simulink model "Intergration"  (R2018b)
settings: Solver=FixedStepDiscrete  StartTime=0.0  StopTime=inf  FixedStep=0.005  RelTol=1e-3
PostLoadFcn:
  | if any(exist('dsrtsu_mdlpostloadfcn', 'file') ~= 0), dsrtsu_mdlpostloadfcn('Execute', bdroot); end
values from neighbouring files (symbols this model uses):
  P_x165_On = 1.0    [CAN_Tx.sldd]
  P_x242_On = 1.0    [CAN_Tx.sldd]
  P_x246_On = 1.0    [CAN_Tx.sldd]
libraries: rtican x112, simulink x59
(part 30 of 31)

== system Intergration/Radar410_RX/Subsystem41/Subsystem6 ==
  In1 : Inport
  Bus Creator : BusCreator  Inputs=20  OutDataTypeStr=Bus: Obj_Data  NonVirtualBus=on
      settings: InheritFromInputs=off
  Bus Selector : BusSelector  OutputSignals=FRS_P1_06_Msg_CheckSum,FRS_P1_06_Msg_AliveCounter,FRS_P1_06_Obj_ExstProb,FRS_P1_06_Obj_XVelRel_Stdev,FRS_P1_06_Obj_XAccRel,FRS_P1_06_Obj_ObstacleProb,FRS_P1_06_Obj_MotionPattern,FRS_P1_06_Obj_YPos_Stdev,FRS_P1_06_Obj_ValidFlag,FRS_P1_06_Obj_XPos_Stdev,FRS_P1_06_Obj_UpdateFlag,FRS_P1_06_Obj_ID,FRS_P2_06_Msg_CheckSum,FRS_P2_06_Msg_AliveCounter,FRS_P2_06_Obj_MeasFlag,FRS_P2_06_Obj_YVelRel,FRS_P2_06_Obj_Type,FRS_P2_06_Obj_XPos,FRS_P2_06_Obj_YPos,FRS_P2_06_Obj_XVelRel
  Data Type Conversion{,1..19} (20 alike) : DataTypeConversion  OutDataTypeStr=single
  Out1 : Outport  OutDataTypeStr=Bus: Obj_Data
  wires:
  Data Type Conversion19/1 -> Bus Creator/20
  Data Type Conversion14/1 -> Bus Creator/15
  Data Type Conversion8/1 -> Bus Creator/9
  Data Type Conversion7/1 -> Bus Creator/8
  Data Type Conversion3/1 -> Bus Creator/4
  Data Type Conversion4/1 -> Bus Creator/5
  Data Type Conversion1/1 -> Bus Creator/2
  Data Type Conversion13/1 -> Bus Creator/14
  Data Type Conversion2/1 -> Bus Creator/3
  Data Type Conversion/1 -> Bus Creator/1
  Bus Creator/1 -> Out1/1
  In1/1 -> Bus Selector/1
  Bus Selector/20 -> Data Type Conversion19/1  "<FRS_P2_06_Obj_XVelRel>"
  Bus Selector/18 -> Data Type Conversion17/1  "<FRS_P2_06_Obj_XPos>"
  Bus Selector/19 -> Data Type Conversion18/1  "<FRS_P2_06_Obj_YPos>"
  Bus Selector/14 -> Data Type Conversion13/1  "<FRS_P2_06_Msg_AliveCounter>"
  Data Type Conversion10/1 -> Bus Creator/11
  Bus Selector/10 -> Data Type Conversion9/1  "<FRS_P1_06_Obj_XPos_Stdev>"
  Bus Selector/17 -> Data Type Conversion16/1  "<FRS_P2_06_Obj_Type>"
  Bus Selector/9 -> Data Type Conversion8/1  "<FRS_P1_06_Obj_ValidFlag>"
  Data Type Conversion16/1 -> Bus Creator/17
  Bus Selector/12 -> Data Type Conversion11/1  "<FRS_P1_06_Obj_ID>"
  Data Type Conversion6/1 -> Bus Creator/7
  Bus Selector/16 -> Data Type Conversion15/1  "<FRS_P2_06_Obj_YVelRel>"
  Data Type Conversion17/1 -> Bus Creator/18
  Bus Selector/11 -> Data Type Conversion10/1  "<FRS_P1_06_Obj_UpdateFlag>"
  Data Type Conversion18/1 -> Bus Creator/19
  Bus Selector/6 -> Data Type Conversion5/1  "<FRS_P1_06_Obj_ObstacleProb>"
  Data Type Conversion9/1 -> Bus Creator/10
  Bus Selector/7 -> Data Type Conversion6/1  "<FRS_P1_06_Obj_MotionPattern>"
  Bus Selector/4 -> Data Type Conversion3/1  "<FRS_P1_06_Obj_XVelRel_Stdev>"
  Data Type Conversion5/1 -> Bus Creator/6
  Data Type Conversion11/1 -> Bus Creator/12
  Bus Selector/2 -> Data Type Conversion1/1  "<FRS_P1_06_Msg_AliveCounter>"
  Bus Selector/13 -> Data Type Conversion12/1  "<FRS_P2_06_Msg_CheckSum>"
  Bus Selector/3 -> Data Type Conversion2/1  "<FRS_P1_06_Obj_ExstProb>"
  Bus Selector/15 -> Data Type Conversion14/1  "<FRS_P2_06_Obj_MeasFlag>"
  Bus Selector/1 -> Data Type Conversion/1  "<FRS_P1_06_Msg_CheckSum>"
  Data Type Conversion15/1 -> Bus Creator/16
  Bus Selector/8 -> Data Type Conversion7/1  "<FRS_P1_06_Obj_YPos_Stdev>"
  Bus Selector/5 -> Data Type Conversion4/1  "<FRS_P1_06_Obj_XAccRel>"
  Data Type Conversion12/1 -> Bus Creator/13

== system Intergration/Radar410_RX/Subsystem41/Subsystem7 ==
  In1 : Inport
  Bus Creator : BusCreator  Inputs=20  OutDataTypeStr=Bus: Obj_Data  NonVirtualBus=on
      settings: InheritFromInputs=off
  Bus Selector : BusSelector  OutputSignals=FRS_P1_07_Msg_CheckSum,FRS_P1_07_Msg_AliveCounter,FRS_P1_07_Obj_ExstProb,FRS_P1_07_Obj_XVelRel_Stdev,FRS_P1_07_Obj_XAccRel,FRS_P1_07_Obj_ObstacleProb,FRS_P1_07_Obj_MotionPattern,FRS_P1_07_Obj_YPos_Stdev,FRS_P1_07_Obj_ValidFlag,FRS_P1_07_Obj_XPos_Stdev,FRS_P1_07_Obj_UpdateFlag,FRS_P1_07_Obj_ID,FRS_P2_07_Msg_CheckSum,FRS_P2_07_Msg_AliveCounter,FRS_P2_07_Obj_MeasFlag,FRS_P2_07_Obj_YVelRel,FRS_P2_07_Obj_Type,FRS_P2_07_Obj_XPos,FRS_P2_07_Obj_YPos,FRS_P2_07_Obj_XVelRel
  Data Type Conversion{,1..19} (20 alike) : DataTypeConversion  OutDataTypeStr=single
  Out1 : Outport  OutDataTypeStr=Bus: Obj_Data
  wires:
  Data Type Conversion12/1 -> Bus Creator/13
  Bus Selector/5 -> Data Type Conversion4/1  "<FRS_P1_07_Obj_XAccRel>"
  Bus Selector/8 -> Data Type Conversion7/1  "<FRS_P1_07_Obj_YPos_Stdev>"
  Data Type Conversion15/1 -> Bus Creator/16
  Bus Selector/1 -> Data Type Conversion/1  "<FRS_P1_07_Msg_CheckSum>"
  Bus Selector/15 -> Data Type Conversion14/1  "<FRS_P2_07_Obj_MeasFlag>"
  Bus Selector/3 -> Data Type Conversion2/1  "<FRS_P1_07_Obj_ExstProb>"
  Bus Selector/13 -> Data Type Conversion12/1  "<FRS_P2_07_Msg_CheckSum>"
  Bus Selector/2 -> Data Type Conversion1/1  "<FRS_P1_07_Msg_AliveCounter>"
  Data Type Conversion11/1 -> Bus Creator/12
  Data Type Conversion5/1 -> Bus Creator/6
  Bus Selector/4 -> Data Type Conversion3/1  "<FRS_P1_07_Obj_XVelRel_Stdev>"
  Bus Selector/7 -> Data Type Conversion6/1  "<FRS_P1_07_Obj_MotionPattern>"
  Data Type Conversion9/1 -> Bus Creator/10
  Bus Selector/6 -> Data Type Conversion5/1  "<FRS_P1_07_Obj_ObstacleProb>"
  Data Type Conversion18/1 -> Bus Creator/19
  Bus Selector/11 -> Data Type Conversion10/1  "<FRS_P1_07_Obj_UpdateFlag>"
  Data Type Conversion17/1 -> Bus Creator/18
  Bus Selector/16 -> Data Type Conversion15/1  "<FRS_P2_07_Obj_YVelRel>"
  Data Type Conversion6/1 -> Bus Creator/7
  Bus Selector/12 -> Data Type Conversion11/1  "<FRS_P1_07_Obj_ID>"
  Data Type Conversion16/1 -> Bus Creator/17
  Bus Selector/9 -> Data Type Conversion8/1  "<FRS_P1_07_Obj_ValidFlag>"
  Bus Selector/17 -> Data Type Conversion16/1  "<FRS_P2_07_Obj_Type>"
  Bus Selector/10 -> Data Type Conversion9/1  "<FRS_P1_07_Obj_XPos_Stdev>"
  Data Type Conversion10/1 -> Bus Creator/11
  Bus Selector/14 -> Data Type Conversion13/1  "<FRS_P2_07_Msg_AliveCounter>"
  Bus Selector/19 -> Data Type Conversion18/1  "<FRS_P2_07_Obj_YPos>"
  Bus Selector/18 -> Data Type Conversion17/1  "<FRS_P2_07_Obj_XPos>"
  Bus Selector/20 -> Data Type Conversion19/1  "<FRS_P2_07_Obj_XVelRel>"
  In1/1 -> Bus Selector/1
  Bus Creator/1 -> Out1/1
  Data Type Conversion/1 -> Bus Creator/1
  Data Type Conversion2/1 -> Bus Creator/3
  Data Type Conversion13/1 -> Bus Creator/14
  Data Type Conversion1/1 -> Bus Creator/2
  Data Type Conversion4/1 -> Bus Creator/5
  Data Type Conversion3/1 -> Bus Creator/4
  Data Type Conversion7/1 -> Bus Creator/8
  Data Type Conversion8/1 -> Bus Creator/9
  Data Type Conversion14/1 -> Bus Creator/15
  Data Type Conversion19/1 -> Bus Creator/20

== system Intergration/Radar410_RX/Subsystem41/Subsystem8 ==
  In1 : Inport
  Bus Creator : BusCreator  Inputs=20  OutDataTypeStr=Bus: Obj_Data  NonVirtualBus=on
      settings: InheritFromInputs=off
  Bus Selector : BusSelector  OutputSignals=FRS_P1_08_Msg_CheckSum,FRS_P1_08_Msg_AliveCounter,FRS_P1_08_Obj_ExstProb,FRS_P1_08_Obj_XVelRel_Stdev,FRS_P1_08_Obj_XAccRel,FRS_P1_08_Obj_ObstacleProb,FRS_P1_08_Obj_MotionPattern,FRS_P1_08_Obj_YPos_Stdev,FRS_P1_08_Obj_ValidFlag,FRS_P1_08_Obj_XPos_Stdev,FRS_P1_08_Obj_UpdateFlag,FRS_P1_08_Obj_ID,FRS_P2_08_Msg_CheckSum,FRS_P2_08_Msg_AliveCounter,FRS_P2_08_Obj_MeasFlag,FRS_P2_08_Obj_YVelRel,FRS_P2_08_Obj_Type,FRS_P2_08_Obj_XPos,FRS_P2_08_Obj_YPos,FRS_P2_08_Obj_XVelRel
  Data Type Conversion{,1..19} (20 alike) : DataTypeConversion  OutDataTypeStr=single
  Out1 : Outport  OutDataTypeStr=Bus: Obj_Data
  wires:
  Data Type Conversion12/1 -> Bus Creator/13
  Bus Selector/5 -> Data Type Conversion4/1  "<FRS_P1_08_Obj_XAccRel>"
  Bus Selector/8 -> Data Type Conversion7/1  "<FRS_P1_08_Obj_YPos_Stdev>"
  Data Type Conversion15/1 -> Bus Creator/16
  Bus Selector/1 -> Data Type Conversion/1  "<FRS_P1_08_Msg_CheckSum>"
  Bus Selector/15 -> Data Type Conversion14/1  "<FRS_P2_08_Obj_MeasFlag>"
  Bus Selector/3 -> Data Type Conversion2/1  "<FRS_P1_08_Obj_ExstProb>"
  Bus Selector/13 -> Data Type Conversion12/1  "<FRS_P2_08_Msg_CheckSum>"
  Bus Selector/2 -> Data Type Conversion1/1  "<FRS_P1_08_Msg_AliveCounter>"
  Data Type Conversion11/1 -> Bus Creator/12
  Data Type Conversion5/1 -> Bus Creator/6
  Bus Selector/4 -> Data Type Conversion3/1  "<FRS_P1_08_Obj_XVelRel_Stdev>"
  Bus Selector/7 -> Data Type Conversion6/1  "<FRS_P1_08_Obj_MotionPattern>"
  Data Type Conversion9/1 -> Bus Creator/10
  Bus Selector/6 -> Data Type Conversion5/1  "<FRS_P1_08_Obj_ObstacleProb>"
  Data Type Conversion18/1 -> Bus Creator/19
  Bus Selector/11 -> Data Type Conversion10/1  "<FRS_P1_08_Obj_UpdateFlag>"
  Data Type Conversion17/1 -> Bus Creator/18
  Bus Selector/16 -> Data Type Conversion15/1  "<FRS_P2_08_Obj_YVelRel>"
  Data Type Conversion6/1 -> Bus Creator/7
  Bus Selector/12 -> Data Type Conversion11/1  "<FRS_P1_08_Obj_ID>"
  Data Type Conversion16/1 -> Bus Creator/17
  Bus Selector/9 -> Data Type Conversion8/1  "<FRS_P1_08_Obj_ValidFlag>"
  Bus Selector/17 -> Data Type Conversion16/1  "<FRS_P2_08_Obj_Type>"
  Bus Selector/10 -> Data Type Conversion9/1  "<FRS_P1_08_Obj_XPos_Stdev>"
  Data Type Conversion10/1 -> Bus Creator/11
  Bus Selector/14 -> Data Type Conversion13/1  "<FRS_P2_08_Msg_AliveCounter>"
  Bus Selector/19 -> Data Type Conversion18/1  "<FRS_P2_08_Obj_YPos>"
  Bus Selector/18 -> Data Type Conversion17/1  "<FRS_P2_08_Obj_XPos>"
  Bus Selector/20 -> Data Type Conversion19/1  "<FRS_P2_08_Obj_XVelRel>"
  In1/1 -> Bus Selector/1
  Bus Creator/1 -> Out1/1
  Data Type Conversion/1 -> Bus Creator/1
  Data Type Conversion2/1 -> Bus Creator/3
  Data Type Conversion13/1 -> Bus Creator/14
  Data Type Conversion1/1 -> Bus Creator/2
  Data Type Conversion4/1 -> Bus Creator/5
  Data Type Conversion3/1 -> Bus Creator/4
  Data Type Conversion7/1 -> Bus Creator/8
  Data Type Conversion8/1 -> Bus Creator/9
  Data Type Conversion14/1 -> Bus Creator/15
  Data Type Conversion19/1 -> Bus Creator/20

== system Intergration/Radar410_RX/Subsystem41/Subsystem9 ==
  In1 : Inport
  Bus Creator : BusCreator  Inputs=20  OutDataTypeStr=Bus: Obj_Data  NonVirtualBus=on
      settings: InheritFromInputs=off
  Bus Selector : BusSelector  OutputSignals=FRS_P1_09_Msg_CheckSum,FRS_P1_09_Msg_AliveCounter,FRS_P1_09_Obj_ExstProb,FRS_P1_09_Obj_XVelRel_Stdev,FRS_P1_09_Obj_XAccRel,FRS_P1_09_Obj_ObstacleProb,FRS_P1_09_Obj_MotionPattern,FRS_P1_09_Obj_YPos_Stdev,FRS_P1_09_Obj_ValidFlag,FRS_P1_09_Obj_XPos_Stdev,FRS_P1_09_Obj_UpdateFlag,FRS_P1_09_Obj_ID,FRS_P2_09_Msg_CheckSum,FRS_P2_09_Msg_AliveCounter,FRS_P2_09_Obj_MeasFlag,FRS_P2_09_Obj_YVelRel,FRS_P2_09_Obj_Type,FRS_P2_09_Obj_XPos,FRS_P2_09_Obj_YPos,FRS_P2_09_Obj_XVelRel
  Data Type Conversion{,1..19} (20 alike) : DataTypeConversion  OutDataTypeStr=single
  Out1 : Outport  OutDataTypeStr=Bus: Obj_Data
  wires:
  Data Type Conversion19/1 -> Bus Creator/20
  Data Type Conversion14/1 -> Bus Creator/15
  Data Type Conversion8/1 -> Bus Creator/9
  Data Type Conversion7/1 -> Bus Creator/8
  Data Type Conversion3/1 -> Bus Creator/4
  Data Type Conversion4/1 -> Bus Creator/5
  Data Type Conversion1/1 -> Bus Creator/2
  Data Type Conversion13/1 -> Bus Creator/14
  Data Type Conversion2/1 -> Bus Creator/3
  Data Type Conversion/1 -> Bus Creator/1
  Bus Creator/1 -> Out1/1
  In1/1 -> Bus Selector/1
  Bus Selector/20 -> Data Type Conversion19/1  "<FRS_P2_09_Obj_XVelRel>"
  Bus Selector/18 -> Data Type Conversion17/1  "<FRS_P2_09_Obj_XPos>"
  Bus Selector/19 -> Data Type Conversion18/1  "<FRS_P2_09_Obj_YPos>"
  Bus Selector/14 -> Data Type Conversion13/1  "<FRS_P2_09_Msg_AliveCounter>"
  Data Type Conversion10/1 -> Bus Creator/11
  Bus Selector/10 -> Data Type Conversion9/1  "<FRS_P1_09_Obj_XPos_Stdev>"
  Bus Selector/17 -> Data Type Conversion16/1  "<FRS_P2_09_Obj_Type>"
  Bus Selector/9 -> Data Type Conversion8/1  "<FRS_P1_09_Obj_ValidFlag>"
  Data Type Conversion16/1 -> Bus Creator/17
  Bus Selector/12 -> Data Type Conversion11/1  "<FRS_P1_09_Obj_ID>"
  Data Type Conversion6/1 -> Bus Creator/7
  Bus Selector/16 -> Data Type Conversion15/1  "<FRS_P2_09_Obj_YVelRel>"
  Data Type Conversion17/1 -> Bus Creator/18
  Bus Selector/11 -> Data Type Conversion10/1  "<FRS_P1_09_Obj_UpdateFlag>"
  Data Type Conversion18/1 -> Bus Creator/19
  Bus Selector/6 -> Data Type Conversion5/1  "<FRS_P1_09_Obj_ObstacleProb>"
  Data Type Conversion9/1 -> Bus Creator/10
  Bus Selector/7 -> Data Type Conversion6/1  "<FRS_P1_09_Obj_MotionPattern>"
  Bus Selector/4 -> Data Type Conversion3/1  "<FRS_P1_09_Obj_XVelRel_Stdev>"
  Data Type Conversion5/1 -> Bus Creator/6
  Data Type Conversion11/1 -> Bus Creator/12
  Bus Selector/2 -> Data Type Conversion1/1  "<FRS_P1_09_Msg_AliveCounter>"
  Bus Selector/13 -> Data Type Conversion12/1  "<FRS_P2_09_Msg_CheckSum>"
  Bus Selector/3 -> Data Type Conversion2/1  "<FRS_P1_09_Obj_ExstProb>"
  Bus Selector/15 -> Data Type Conversion14/1  "<FRS_P2_09_Obj_MeasFlag>"
  Bus Selector/1 -> Data Type Conversion/1  "<FRS_P1_09_Msg_CheckSum>"
  Data Type Conversion15/1 -> Bus Creator/16
  Bus Selector/8 -> Data Type Conversion7/1  "<FRS_P1_09_Obj_YPos_Stdev>"
  Bus Selector/5 -> Data Type Conversion4/1  "<FRS_P1_09_Obj_XAccRel>"
  Data Type Conversion12/1 -> Bus Creator/13

== system Intergration/TX/Adapter_Tx/calc_0x165 ==
  <EngineTorqReq> : Inport
  <EngineTorqReqSt> : Inport  Port=2
  Bus Creator3 : BusCreator  Inputs=2  OutDataTypeStr=Bus: x165  NonVirtualBus=on
      settings: InheritFromInputs=off
  EngineTorqReq : Constant  Value=0  OutDataTypeStr=single
  EngineTorqReqSt : Constant  Value=0  OutDataTypeStr=boolean
  P_x165_On : Constant  Value=P_x165_On
  Switch : Switch  Criteria=u2 > Threshold  OutDataTypeStr=Inherit: Inherit via back propagation
  Switch1 : Switch  Criteria=u2 > Threshold  OutDataTypeStr=Inherit: Inherit via back propagation
  COM_x165_st : Outport
  wires:
  Switch1/1 -> Bus Creator3/2  "EngineTorqReq"
  P_x165_On/1 -> Switch/2, Switch1/2
  EngineTorqReq/1 -> Switch1/3
  <EngineTorqReq>/1 -> Switch1/1
  <EngineTorqReqSt>/1 -> Switch/1
  Switch/1 -> Bus Creator3/1  "EngineTorqReqSt"
  Bus Creator3/1 -> COM_x165_st/1  "COM_x165_st"
  EngineTorqReqSt/1 -> Switch/3

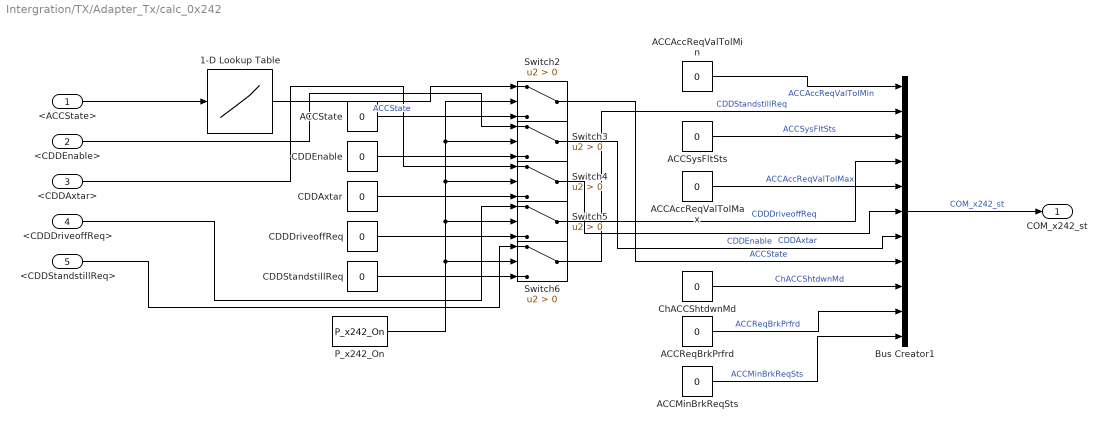
== system Intergration/TX/Adapter_Tx/calc_0x242 ==
  <ACCState> : Inport
  <CDDEnable> : Inport  Port=2
  <CDDAxtar> : Inport  Port=3
  <CDDDriveoffReq> : Inport  Port=4
  <CDDStandstillReq> : Inport  Port=5
  1-D Lookup Table : Lookup_n-D  NumberOfTableDimensions=1  BreakpointsForDimension1=[0,1,2,3,4]  Table=[0,1,2,5,3]  InternalRulePriority=Speed  RndMeth=Simplest  InputSameDT=on
  ACCAccReqValTolMax : Constant  Value=0  OutDataTypeStr=single
  ACCAccReqValTolMin : Constant  Value=0  OutDataTypeStr=single
  ACCMinBrkReqSts : Constant  Value=0  OutDataTypeStr=boolean
  ACCReqBrkPrfrd : Constant  Value=0  OutDataTypeStr=boolean
  ACCState : Constant  Value=0  OutDataTypeStr=single
  ACCSysFltSts : Constant  Value=0  OutDataTypeStr=single
  Bus Creator1 : BusCreator  Inputs=11  OutDataTypeStr=Bus: x242  NonVirtualBus=on
  CDDAxtar : Constant  Value=0  OutDataTypeStr=single
  CDDDriveoffReq : Constant  Value=0  OutDataTypeStr=boolean
  CDDEnable : Constant  Value=0  OutDataTypeStr=boolean
  CDDStandstillReq : Constant  Value=0  OutDataTypeStr=boolean
  ChACCShtdwnMd : Constant  Value=0  OutDataTypeStr=single
  P_x242_On : Constant  Value=P_x242_On
  Switch{2..6} (5 alike) : Switch  Criteria=u2 > Threshold  OutDataTypeStr=Inherit: Inherit via back propagation
  COM_x242_st : Outport
  wires:
  Switch2/1 -> Bus Creator1/8  "ACCState"
  CDDStandstillReq/1 -> Switch6/3
  ACCState/1 -> Switch2/3
  <CDDStandstillReq>/1 -> Switch6/1
  P_x242_On/1 -> Switch5/2, Switch4/2, Switch2/2, Switch3/2, Switch6/2
  CDDDriveoffReq/1 -> Switch5/3
  ACCAccReqValTolMax/1 -> Bus Creator1/5  "ACCAccReqValTolMax"
  CDDAxtar/1 -> Switch4/3
  CDDEnable/1 -> Switch3/3
  <ACCState>/1 -> 1-D Lookup Table/1
  Switch3/1 -> Bus Creator1/7  "CDDEnable"
  ACCReqBrkPrfrd/1 -> Bus Creator1/10  "ACCReqBrkPrfrd"
  ChACCShtdwnMd/1 -> Bus Creator1/9  "ChACCShtdwnMd"
  Switch4/1 -> Bus Creator1/6  "CDDAxtar"
  Switch6/1 -> Bus Creator1/2  "CDDStandstillReq"
  ACCSysFltSts/1 -> Bus Creator1/3  "ACCSysFltSts"
  ACCMinBrkReqSts/1 -> Bus Creator1/11  "ACCMinBrkReqSts"
  Switch5/1 -> Bus Creator1/4  "CDDDriveoffReq"
  <CDDDriveoffReq>/1 -> Switch5/1
  ACCAccReqValTolMin/1 -> Bus Creator1/1  "ACCAccReqValTolMin"
  1-D Lookup Table/1 -> Switch2/1  "ACCState"
  Bus Creator1/1 -> COM_x242_st/1  "COM_x242_st"
  <CDDAxtar>/1 -> Switch4/1
  <CDDEnable>/1 -> Switch3/1

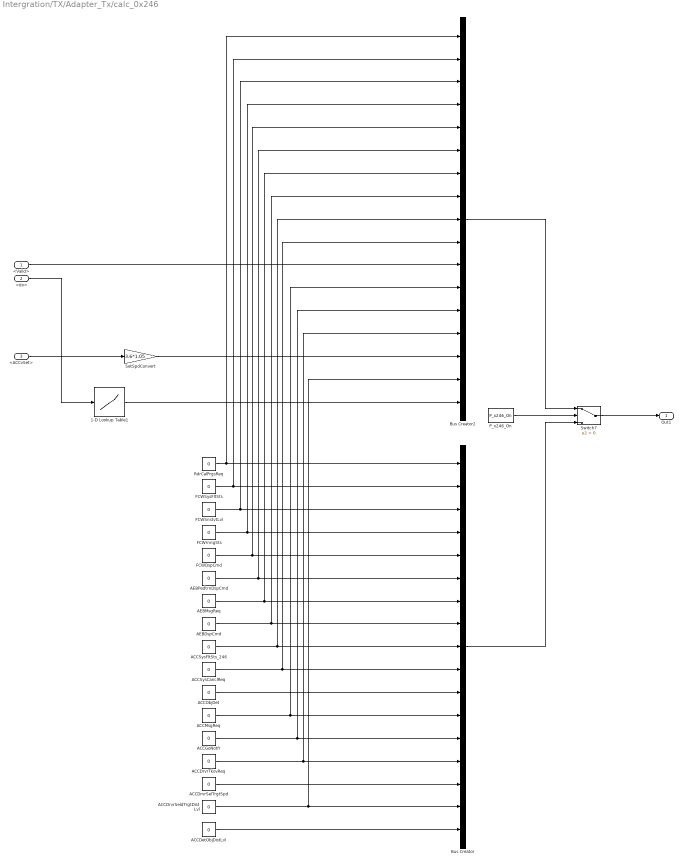
== system Intergration/TX/Adapter_Tx/calc_0x246 ==
  <Valid> : Inport
  <dx> : Inport  Port=2
  <ACCvSet> : Inport  Port=3
  1-D Lookup Table1 : Lookup_n-D  NumberOfTableDimensions=1  LookupTableObject=''  BreakpointsForDimension1=[5,10,20,30,40]  BreakpointsForDimension1FirstPoint=10  BreakpointsForDimension2FirstPoint=10  BreakpointsForDimension1Spacing=12  BreakpointsForDimension2Spacing=12  IndexSearchMethod=Linear search  Table=[1,2,3,4,5]  InterpMethod=Flat  InternalRulePriority=Speed  RndMeth=Simplest  InputSameDT=on
  ACCDetObjDistLvl : Constant  Value=0  OutDataTypeStr=single
  ACCDrvrSelTrgtSpd : Constant  Value=0  OutDataTypeStr=single
  ACCDrvrSeldTrgtDistLvl : Constant  Value=0  OutDataTypeStr=single
  ACCDrvrTkovReq : Constant  Value=0  OutDataTypeStr=boolean
  ACCGoNotfr : Constant  Value=0  OutDataTypeStr=boolean
  ACCMsgReq : Constant  Value=0  OutDataTypeStr=single
  ACCObjDet : Constant  Value=0  OutDataTypeStr=boolean
  ACCSysCanclReq : Constant  Value=0  OutDataTypeStr=single
  ACCSysFltSts_246 : Constant  Value=0  OutDataTypeStr=single
  AEBDspCmd : Constant  Value=0  OutDataTypeStr=single
  AEBMsgReq : Constant  Value=0  OutDataTypeStr=single
  AEBPedtrnDspCmd : Constant  Value=0  OutDataTypeStr=single
  Bus Creator : BusCreator  Inputs=17  OutDataTypeStr=Bus: x246  NonVirtualBus=on
      settings: InheritFromInputs=off
  Bus Creator2 : BusCreator  Inputs=17  OutDataTypeStr=Bus: x246  NonVirtualBus=on
      settings: InheritFromInputs=off
  FCWDspCmd : Constant  Value=0  OutDataTypeStr=single
  FCWSnstvtLvl : Constant  Value=0  OutDataTypeStr=single
  FCWSysFltSts : Constant  Value=0  OutDataTypeStr=single
  FCWrnngSts : Constant  Value=0  OutDataTypeStr=single
  P_x246_On : Constant  Value=P_x246_On
  RdrCalPrgsReq : Constant  Value=0  OutDataTypeStr=single
  SetSpdConvert : Gain  Gain=3.6*1.05
  Switch7 : Switch  Criteria=u2 > Threshold
  Out1 : Outport
  wires:
  ACCDrvrSeldTrgtDistLvl/1 -> Bus Creator2/16, Bus Creator/16
  ACCSysCanclReq/1 -> Bus Creator2/10, Bus Creator/10
  FCWDspCmd/1 -> Bus Creator2/5, Bus Creator/5
  ACCSysFltSts_246/1 -> Bus Creator2/9, Bus Creator/9
  FCWrnngSts/1 -> Bus Creator2/4, Bus Creator/4
  SetSpdConvert/1 -> Bus Creator2/15
  Bus Creator2/1 -> Switch7/1
  Bus Creator/1 -> Switch7/3
  ACCDetObjDistLvl/1 -> Bus Creator/17
  <ACCvSet>/1 -> SetSpdConvert/1
  FCWSysFltSts/1 -> Bus Creator2/2, Bus Creator/2
  RdrCalPrgsReq/1 -> Bus Creator2/1, Bus Creator/1
  ACCGoNotfr/1 -> Bus Creator2/13, Bus Creator/13
  ACCDrvrSelTrgtSpd/1 -> Bus Creator/15
  <Valid>/1 -> Bus Creator2/11
  AEBMsgReq/1 -> Bus Creator2/7, Bus Creator/7
  AEBDspCmd/1 -> Bus Creator2/8, Bus Creator/8
  ACCDrvrTkovReq/1 -> Bus Creator2/14, Bus Creator/14
  <dx>/1 -> 1-D Lookup Table1/1
  FCWSnstvtLvl/1 -> Bus Creator2/3, Bus Creator/3
  ACCMsgReq/1 -> Bus Creator2/12, Bus Creator/12
  ACCObjDet/1 -> Bus Creator/11
  P_x246_On/1 -> Switch7/2
  AEBPedtrnDspCmd/1 -> Bus Creator2/6, Bus Creator/6
  1-D Lookup Table1/1 -> Bus Creator2/17
  Switch7/1 -> Out1/1

== system Intergration/TX/Adapter_Tx/calc_0x255 ==
  ACCvSet : Inport
  ACCState : Inport  Port=2
  dx : Inport  Port=3
  dy : Inport  Port=4
  Type : Inport  Port=5
  ACC_Error : Constant  Value=0  OutDataTypeStr=single
  ACC_Passive_Res : Constant  Value=0  OutDataTypeStr=single
  ACC_Tip : Constant  Value=0  OutDataTypeStr=single
  Bus Creator : BusCreator  Inputs=9  OutDataTypeStr=Bus: x255  NonVirtualBus=on
      settings: InheritFromInputs=off
  TimeGapRes : Constant  Value=0  OutDataTypeStr=single
  Out1 : Outport
  wires:
  dy/1 -> Bus Creator/1
  dx/1 -> Bus Creator/2
  Type/1 -> Bus Creator/3
  ACC_Tip/1 -> Bus Creator/4
  ACCState/1 -> Bus Creator/5
  ACC_Passive_Res/1 -> Bus Creator/6
  ACC_Error/1 -> Bus Creator/7
  TimeGapRes/1 -> Bus Creator/8
  ACCvSet/1 -> Bus Creator/9
  Bus Creator/1 -> Out1/1

== system Intergration/TX/ESC_DA_MESSAGE_0x127/RollingCounter1 ==
  Add2 : Sum
  Constant5 : Constant
  Constant6 : Constant  Value=-1
  Delay : Delay  DelayLength=1
  Switch : Switch  Criteria=u2 > Threshold  Threshold=14
  RC : Outport
  wires:
  Constant6/1 -> Switch/1
  Switch/1 -> Add2/2
  Delay/1 -> RC/1, Switch/3, Switch/2
  Add2/1 -> Delay/1
  Constant5/1 -> Add2/1

== system Intergration/TX/ESC_DA_MESSAGE_0x127/Subsystem ==
  NoBrakeForce : Inport
  ABP_available : Inport  Port=2
  AEB_available : Inport  Port=3
  Add : Sum  Inputs=+++
  Bitwise Operator1 : simulink/Logic and Bit Operations/Bitwise Operator  logicop=AND  UseBitMask=on  BitMask=bin2dec('00010000')  BitMaskRealWorld=Stored Integer
  Bitwise Operator2 : simulink/Logic and Bit Operations/Bitwise Operator  logicop=AND  UseBitMask=on  BitMask=bin2dec('00000100')  BitMaskRealWorld=Stored Integer
  Bitwise Operator3 : simulink/Logic and Bit Operations/Bitwise Operator  logicop=AND  UseBitMask=on  BitMask=bin2dec('10000000')  BitMaskRealWorld=Stored Integer
  Data Type Conversion1 : DataTypeConversion  OutDataTypeStr=uint8
  Data Type Conversion2 : DataTypeConversion  OutDataTypeStr=uint8
  Data Type Conversion3 : DataTypeConversion  OutDataTypeStr=uint8
  Shift Arithmetic1 : ArithShift  BitShiftNumber=4  BitShiftDirection=Left
  Shift Arithmetic2 : ArithShift  BitShiftNumber=7  BitShiftDirection=Left
  Shift Arithmetic3 : ArithShift  BitShiftNumber=2  BitShiftDirection=Left
  Byte0 : Outport
  wires:
  Bitwise Operator1/1 -> Add/2
  Data Type Conversion2/1 -> Shift Arithmetic3/1
  Shift Arithmetic2/1 -> Bitwise Operator3/1
  Data Type Conversion3/1 -> Shift Arithmetic2/1
  Data Type Conversion1/1 -> Shift Arithmetic1/1
  Shift Arithmetic3/1 -> Bitwise Operator2/1
  Bitwise Operator3/1 -> Add/1
  Add/1 -> Byte0/1
  Shift Arithmetic1/1 -> Bitwise Operator1/1
  Bitwise Operator2/1 -> Add/3
  NoBrakeForce/1 -> Data Type Conversion2/1
  ABP_available/1 -> Data Type Conversion1/1
  AEB_available/1 -> Data Type Conversion3/1

== system Intergration/TX/ESC_DA_MESSAGE_0x127/Subsystem1 ==
  ABA_available : Inport
  AWB_available : Inport  Port=2
  VehSdslStsHSC2 : Inport  Port=3
  Add : Sum  Inputs=+++
  Bitwise Operator1 : simulink/Logic and Bit Operations/Bitwise Operator  logicop=AND  UseBitMask=on  BitMask=bin2dec('00001000')  BitMaskRealWorld=Stored Integer
  Bitwise Operator2 : simulink/Logic and Bit Operations/Bitwise Operator  logicop=AND  UseBitMask=on  BitMask=bin2dec('11000000')  BitMaskRealWorld=Stored Integer
  Bitwise Operator3 : simulink/Logic and Bit Operations/Bitwise Operator  logicop=AND  UseBitMask=on  BitMask=bin2dec('00000010')  BitMaskRealWorld=Stored Integer
  Data Type Conversion1 : DataTypeConversion  OutDataTypeStr=uint8
  Data Type Conversion2 : DataTypeConversion  OutDataTypeStr=uint8
  Data Type Conversion3 : DataTypeConversion  OutDataTypeStr=uint8
  Shift Arithmetic1 : ArithShift  BitShiftNumber=3  BitShiftDirection=Left
  Shift Arithmetic2 : ArithShift  BitShiftNumber=1  BitShiftDirection=Left
  Shift Arithmetic3 : ArithShift  BitShiftNumber=6  BitShiftDirection=Left
  Byte1 : Outport
  wires:
  Shift Arithmetic3/1 -> Bitwise Operator2/1
  Shift Arithmetic1/1 -> Bitwise Operator1/1
  ABA_available/1 -> Data Type Conversion3/1
  VehSdslStsHSC2/1 -> Data Type Conversion2/1
  Bitwise Operator1/1 -> Add/2
  Data Type Conversion3/1 -> Shift Arithmetic2/1
  Shift Arithmetic2/1 -> Bitwise Operator3/1
  Bitwise Operator2/1 -> Add/1
  Data Type Conversion1/1 -> Shift Arithmetic1/1
  Data Type Conversion2/1 -> Shift Arithmetic3/1
  Bitwise Operator3/1 -> Add/3
  Add/1 -> Byte1/1
  AWB_available/1 -> Data Type Conversion1/1

== system Intergration/TX/ESC_DA_MESSAGE_0x127/Subsystem2 ==
  In1 : Inport
  Bitwise Operator2 : simulink/Logic and Bit Operations/Bitwise Operator  logicop=AND  UseBitMask=on  BitMask=bin2dec('00001111')  BitMaskRealWorld=Stored Integer
  Data Type Conversion1 : DataTypeConversion  OutDataTypeStr=uint8
  Byte6 : Outport
  wires:
  In1/1 -> Data Type Conversion1/1
  Bitwise Operator2/1 -> Byte6/1
  Data Type Conversion1/1 -> Bitwise Operator2/1

== system Intergration/TX/ESC_FrontWheelSpeedKPH_0x123/RollingCounter1 ==
  Add2 : Sum
  Constant5 : Constant
  Constant6 : Constant  Value=-1
  Delay : Delay  DelayLength=1
  Switch : Switch  Criteria=u2 > Threshold  Threshold=14
  RC : Outport
  wires:
  Constant6/1 -> Switch/1
  Switch/1 -> Add2/2
  Delay/1 -> RC/1, Switch/3, Switch/2
  Add2/1 -> Delay/1
  Constant5/1 -> Add2/1

== system Intergration/TX/ESC_FrontWheelSpeedKPH_0x123/Subsystem ==
  <WhlGndVelLDrvn_Radar> : Inport
  Bitwise Operator1 : simulink/Logic and Bit Operations/Bitwise Operator  logicop=AND  UseBitMask=on  BitMask=bin2dec('11111111')  BitMaskRealWorld=Stored Integer
  Constant : Constant  Value=0.05625
  Constant1 : Constant  Value=0.05625
  Data Type Conversion1 : DataTypeConversion  OutDataTypeStr=uint16
  Data Type Conversion2 : DataTypeConversion  OutDataTypeStr=uint8
  Divide : Product  Inputs=*/
  Multiply : Product
  Shift Arithmetic1 : ArithShift  BitShiftNumber=5  BitShiftDirection=Right
  Out1 : Outport
  Byte0 : Outport  Port=2
  Output : Outport  Port=3
  wires:
  Bitwise Operator1/1 -> Data Type Conversion2/1
  Shift Arithmetic1/1 -> Bitwise Operator1/1
  Divide/1 -> Data Type Conversion1/1
  Constant/1 -> Divide/2
  Constant1/1 -> Multiply/1
  Data Type Conversion1/1 -> Output/1, Multiply/2, Shift Arithmetic1/1
  <WhlGndVelLDrvn_Radar>/1 -> Divide/1
  Multiply/1 -> Out1/1
  Data Type Conversion2/1 -> Byte0/1

== system Intergration/TX/ESC_FrontWheelSpeedKPH_0x123/Subsystem1 ==
  In1 : Inport
  <LDrvnWhlRotlDircn> : Inport  Port=2
  Add : Sum
  Bitwise Operator1 : simulink/Logic and Bit Operations/Bitwise Operator  logicop=AND  UseBitMask=on  BitMask=bin2dec('00000110')  BitMaskRealWorld=Stored Integer
  Bitwise Operator2 : simulink/Logic and Bit Operations/Bitwise Operator  logicop=AND  UseBitMask=on  BitMask=bin2dec('11111000')  BitMaskRealWorld=Stored Integer
  Data Type Conversion1 : DataTypeConversion  OutDataTypeStr=uint8
  Data Type Conversion2 : DataTypeConversion  OutDataTypeStr=uint8
  Shift Arithmetic1 : ArithShift  BitShiftNumber=1  BitShiftDirection=Left
  Shift Arithmetic2 : ArithShift  BitShiftNumber=3  BitShiftDirection=Left
  Byte1 : Outport
  wires:
  <LDrvnWhlRotlDircn>/1 -> Data Type Conversion1/1
  Bitwise Operator2/1 -> Data Type Conversion2/1
  Data Type Conversion1/1 -> Shift Arithmetic1/1
  Bitwise Operator1/1 -> Add/1
  Shift Arithmetic1/1 -> Bitwise Operator1/1
  Add/1 -> Byte1/1
  Shift Arithmetic2/1 -> Bitwise Operator2/1
  In1/1 -> Shift Arithmetic2/1
  Data Type Conversion2/1 -> Add/2

== system Intergration/TX/ESC_FrontWheelSpeedKPH_0x123/Subsystem2 ==
  <WhlGndVelLDrvn_Radar> : Inport
  Bitwise Operator1 : simulink/Logic and Bit Operations/Bitwise Operator  logicop=AND  UseBitMask=on  BitMask=bin2dec('11111111')  BitMaskRealWorld=Stored Integer
  Constant : Constant  Value=0.05625
  Constant1 : Constant  Value=0.05625
  Data Type Conversion1 : DataTypeConversion  OutDataTypeStr=uint16
  Data Type Conversion2 : DataTypeConversion  OutDataTypeStr=uint8
  Divide : Product  Inputs=*/
  Multiply : Product
  Shift Arithmetic1 : ArithShift  BitShiftNumber=5  BitShiftDirection=Right
  Out1 : Outport
  Byte2 : Outport  Port=2
  Output : Outport  Port=3
  wires:
  Bitwise Operator1/1 -> Data Type Conversion2/1
  Shift Arithmetic1/1 -> Bitwise Operator1/1
  Divide/1 -> Data Type Conversion1/1
  Constant/1 -> Divide/2
  Constant1/1 -> Multiply/1
  Data Type Conversion1/1 -> Output/1, Multiply/2, Shift Arithmetic1/1
  <WhlGndVelLDrvn_Radar>/1 -> Divide/1
  Multiply/1 -> Out1/1
  Data Type Conversion2/1 -> Byte2/1

== system Intergration/TX/ESC_FrontWheelSpeedKPH_0x123/Subsystem3 ==
  In1 : Inport
  <LDrvnWhlRotlDircn> : Inport  Port=2
  Add : Sum
  Bitwise Operator1 : simulink/Logic and Bit Operations/Bitwise Operator  logicop=AND  UseBitMask=on  BitMask=bin2dec('00000110')  BitMaskRealWorld=Stored Integer
  Bitwise Operator2 : simulink/Logic and Bit Operations/Bitwise Operator  logicop=AND  UseBitMask=on  BitMask=bin2dec('11111000')  BitMaskRealWorld=Stored Integer
  Data Type Conversion1 : DataTypeConversion  OutDataTypeStr=uint8
  Data Type Conversion2 : DataTypeConversion  OutDataTypeStr=uint8
  Shift Arithmetic1 : ArithShift  BitShiftNumber=1  BitShiftDirection=Left
  Shift Arithmetic2 : ArithShift  BitShiftNumber=3  BitShiftDirection=Left
  Byte3 : Outport
  wires:
  <LDrvnWhlRotlDircn>/1 -> Data Type Conversion1/1
  Bitwise Operator2/1 -> Data Type Conversion2/1
  Data Type Conversion1/1 -> Shift Arithmetic1/1
  Bitwise Operator1/1 -> Add/1
  Shift Arithmetic1/1 -> Bitwise Operator1/1
  Add/1 -> Byte3/1
  Shift Arithmetic2/1 -> Bitwise Operator2/1
  In1/1 -> Shift Arithmetic2/1
  Data Type Conversion2/1 -> Add/2

== system Intergration/TX/ESC_FrontWheelSpeedKPH_0x123/Subsystem4 ==
  In1 : Inport
  Bitwise Operator2 : simulink/Logic and Bit Operations/Bitwise Operator  logicop=AND  UseBitMask=on  BitMask=bin2dec('00001111')  BitMaskRealWorld=Stored Integer
  Data Type Conversion1 : DataTypeConversion  OutDataTypeStr=uint8
  Byte6 : Outport
  wires:
  In1/1 -> Data Type Conversion1/1
  Bitwise Operator2/1 -> Byte6/1
  Data Type Conversion1/1 -> Bitwise Operator2/1

== system Intergration/TX/ESC_RearWheelSpeedKPH_0x124/RollingCounter1 ==
  Add2 : Sum
  Constant5 : Constant
  Constant6 : Constant  Value=-1
  Delay : Delay  DelayLength=1
  Switch : Switch  Criteria=u2 > Threshold  Threshold=14
  RC : Outport
  wires:
  Constant6/1 -> Switch/1
  Switch/1 -> Add2/2
  Delay/1 -> RC/1, Switch/3, Switch/2
  Add2/1 -> Delay/1
  Constant5/1 -> Add2/1

== system Intergration/TX/ESC_RearWheelSpeedKPH_0x124/Subsystem ==
  <WhlGndVelLDrvn_Radar> : Inport
  Bitwise Operator1 : simulink/Logic and Bit Operations/Bitwise Operator  logicop=AND  UseBitMask=on  BitMask=bin2dec('11111111')  BitMaskRealWorld=Stored Integer
  Constant : Constant  Value=0.05625
  Constant1 : Constant  Value=0.05625
  Data Type Conversion1 : DataTypeConversion  OutDataTypeStr=uint16
  Data Type Conversion2 : DataTypeConversion  OutDataTypeStr=uint8
  Divide : Product  Inputs=*/
  Multiply : Product
  Shift Arithmetic1 : ArithShift  BitShiftNumber=5  BitShiftDirection=Right
  Out1 : Outport
  Byte0 : Outport  Port=2
  Output : Outport  Port=3
  wires:
  Bitwise Operator1/1 -> Data Type Conversion2/1
  Shift Arithmetic1/1 -> Bitwise Operator1/1
  Divide/1 -> Data Type Conversion1/1
  Constant/1 -> Divide/2
  Constant1/1 -> Multiply/1
  Data Type Conversion1/1 -> Output/1, Multiply/2, Shift Arithmetic1/1
  <WhlGndVelLDrvn_Radar>/1 -> Divide/1
  Multiply/1 -> Out1/1
  Data Type Conversion2/1 -> Byte0/1

== system Intergration/TX/ESC_RearWheelSpeedKPH_0x124/Subsystem1 ==
  In1 : Inport
  <LDrvnWhlRotlDircn> : Inport  Port=2
  Add : Sum
  Bitwise Operator1 : simulink/Logic and Bit Operations/Bitwise Operator  logicop=AND  UseBitMask=on  BitMask=bin2dec('00000110')  BitMaskRealWorld=Stored Integer
  Bitwise Operator2 : simulink/Logic and Bit Operations/Bitwise Operator  logicop=AND  UseBitMask=on  BitMask=bin2dec('11111000')  BitMaskRealWorld=Stored Integer
  Data Type Conversion1 : DataTypeConversion  OutDataTypeStr=uint8
  Data Type Conversion2 : DataTypeConversion  OutDataTypeStr=uint8
  Shift Arithmetic1 : ArithShift  BitShiftNumber=1  BitShiftDirection=Left
  Shift Arithmetic2 : ArithShift  BitShiftNumber=3  BitShiftDirection=Left
  Byte1 : Outport
  wires:
  <LDrvnWhlRotlDircn>/1 -> Data Type Conversion1/1
  Bitwise Operator2/1 -> Data Type Conversion2/1
  Data Type Conversion1/1 -> Shift Arithmetic1/1
  Bitwise Operator1/1 -> Add/1
  Shift Arithmetic1/1 -> Bitwise Operator1/1
  Add/1 -> Byte1/1
  Shift Arithmetic2/1 -> Bitwise Operator2/1
  In1/1 -> Shift Arithmetic2/1
  Data Type Conversion2/1 -> Add/2

== system Intergration/TX/ESC_RearWheelSpeedKPH_0x124/Subsystem2 ==
  <WhlGndVelLDrvn_Radar> : Inport
  Bitwise Operator1 : simulink/Logic and Bit Operations/Bitwise Operator  logicop=AND  UseBitMask=on  BitMask=bin2dec('11111111')  BitMaskRealWorld=Stored Integer
  Constant : Constant  Value=0.05625
  Constant1 : Constant  Value=0.05625
  Data Type Conversion1 : DataTypeConversion  OutDataTypeStr=uint16
  Data Type Conversion2 : DataTypeConversion  OutDataTypeStr=uint8
  Divide : Product  Inputs=*/
  Multiply : Product
  Shift Arithmetic1 : ArithShift  BitShiftNumber=5  BitShiftDirection=Right
  Out1 : Outport
  Byte2 : Outport  Port=2
  Output : Outport  Port=3
  wires:
  Bitwise Operator1/1 -> Data Type Conversion2/1
  Shift Arithmetic1/1 -> Bitwise Operator1/1
  Divide/1 -> Data Type Conversion1/1
  Constant/1 -> Divide/2
  Constant1/1 -> Multiply/1
  Data Type Conversion1/1 -> Output/1, Multiply/2, Shift Arithmetic1/1
  <WhlGndVelLDrvn_Radar>/1 -> Divide/1
  Multiply/1 -> Out1/1
  Data Type Conversion2/1 -> Byte2/1

== system Intergration/TX/ESC_RearWheelSpeedKPH_0x124/Subsystem3 ==
  In1 : Inport
  <LDrvnWhlRotlDircn> : Inport  Port=2
  Add : Sum
  Bitwise Operator1 : simulink/Logic and Bit Operations/Bitwise Operator  logicop=AND  UseBitMask=on  BitMask=bin2dec('00000110')  BitMaskRealWorld=Stored Integer
  Bitwise Operator2 : simulink/Logic and Bit Operations/Bitwise Operator  logicop=AND  UseBitMask=on  BitMask=bin2dec('11111000')  BitMaskRealWorld=Stored Integer
  Data Type Conversion1 : DataTypeConversion  OutDataTypeStr=uint8
  Data Type Conversion2 : DataTypeConversion  OutDataTypeStr=uint8
  Shift Arithmetic1 : ArithShift  BitShiftNumber=1  BitShiftDirection=Left
  Shift Arithmetic2 : ArithShift  BitShiftNumber=3  BitShiftDirection=Left
  Byte3 : Outport
  wires:
  <LDrvnWhlRotlDircn>/1 -> Data Type Conversion1/1
  Bitwise Operator2/1 -> Data Type Conversion2/1
  Data Type Conversion1/1 -> Shift Arithmetic1/1
  Bitwise Operator1/1 -> Add/1
  Shift Arithmetic1/1 -> Bitwise Operator1/1
  Add/1 -> Byte3/1
  Shift Arithmetic2/1 -> Bitwise Operator2/1
  Data Type Conversion2/1 -> Add/2
  In1/1 -> Shift Arithmetic2/1

== system Intergration/TX/ESC_RearWheelSpeedKPH_0x124/Subsystem4 ==
  In1 : Inport
  Bitwise Operator2 : simulink/Logic and Bit Operations/Bitwise Operator  logicop=AND  UseBitMask=on  BitMask=bin2dec('00001111')  BitMaskRealWorld=Stored Integer
  Data Type Conversion1 : DataTypeConversion  OutDataTypeStr=uint8
  Byte6 : Outport
  wires:
  In1/1 -> Data Type Conversion1/1
  Bitwise Operator2/1 -> Byte6/1
  Data Type Conversion1/1 -> Bitwise Operator2/1

== system Intergration/TX/ESC_Status_0x126/RollingCounter1 ==
  Add2 : Sum
  Constant5 : Constant
  Constant6 : Constant  Value=-1
  Delay : Delay  DelayLength=1
  Switch : Switch  Criteria=u2 > Threshold  Threshold=14
  RC : Outport
  wires:
  Constant6/1 -> Switch/1
  Switch/1 -> Add2/2
  Delay/1 -> RC/1, Switch/3, Switch/2
  Add2/1 -> Delay/1
  Constant5/1 -> Add2/1

== system Intergration/TX/ESC_Status_0x126/Subsystem ==
  <WhlGndVelLDrvn_Radar> : Inport
  Bitwise Operator1 : simulink/Logic and Bit Operations/Bitwise Operator  logicop=AND  UseBitMask=on  BitMask=bin2dec('11111111')  BitMaskRealWorld=Stored Integer
  Constant : Constant  Value=0.05625
  Constant1 : Constant  Value=0.05625
  Data Type Conversion1 : DataTypeConversion  OutDataTypeStr=uint16
  Data Type Conversion2 : DataTypeConversion  OutDataTypeStr=uint8
  Divide : Product  Inputs=*/
  Multiply : Product
  Shift Arithmetic1 : ArithShift  BitShiftNumber=5  BitShiftDirection=Right
  Out1 : Outport
  Byte1 : Outport  Port=2
  Output : Outport  Port=3
  wires:
  Bitwise Operator1/1 -> Data Type Conversion2/1
  Shift Arithmetic1/1 -> Bitwise Operator1/1
  Divide/1 -> Data Type Conversion1/1
  Constant/1 -> Divide/2
  Constant1/1 -> Multiply/1
  Data Type Conversion1/1 -> Output/1, Multiply/2, Shift Arithmetic1/1
  <WhlGndVelLDrvn_Radar>/1 -> Divide/1
  Multiply/1 -> Out1/1
  Data Type Conversion2/1 -> Byte1/1

== system Intergration/TX/ESC_Status_0x126/Subsystem1 ==
  In1 : Inport
  Bitwise Operator2 : simulink/Logic and Bit Operations/Bitwise Operator  logicop=AND  UseBitMask=on  BitMask=bin2dec('11111000')  BitMaskRealWorld=Stored Integer
  Data Type Conversion2 : DataTypeConversion  OutDataTypeStr=uint8
  Shift Arithmetic2 : ArithShift  BitShiftNumber=3  BitShiftDirection=Left
  Byte2 : Outport
  wires:
  In1/1 -> Shift Arithmetic2/1
  Bitwise Operator2/1 -> Data Type Conversion2/1
  Shift Arithmetic2/1 -> Bitwise Operator2/1
  Data Type Conversion2/1 -> Byte2/1

== system Intergration/TX/ESC_Status_0x126/Subsystem4 ==
  In1 : Inport
  Bitwise Operator2 : simulink/Logic and Bit Operations/Bitwise Operator  logicop=AND  UseBitMask=on  BitMask=bin2dec('00001111')  BitMaskRealWorld=Stored Integer
  Data Type Conversion1 : DataTypeConversion  OutDataTypeStr=uint8
  Byte6 : Outport
  wires:
  In1/1 -> Data Type Conversion1/1
  Bitwise Operator2/1 -> Byte6/1
  Data Type Conversion1/1 -> Bitwise Operator2/1

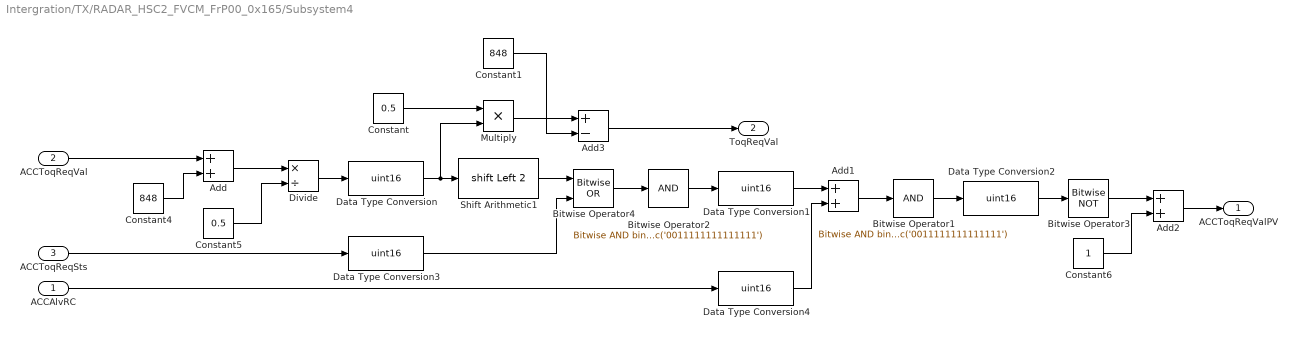
== system Intergration/TX/RADAR_HSC2_FVCM_FrP00_0x165/Subsystem4 ==
  ACCAlvRC : Inport
  ACCToqReqVal : Inport  Port=2
  ACCToqReqSts : Inport  Port=3
  Add : Sum
  Add1 : Sum
  Add2 : Sum
  Add3 : Sum  Inputs=+-
  Bitwise Operator1 : simulink/Logic and Bit Operations/Bitwise Operator  logicop=AND  UseBitMask=on  BitMask=bin2dec('0011111111111111')  BitMaskRealWorld=Stored Integer
  Bitwise Operator2 : simulink/Logic and Bit Operations/Bitwise Operator  logicop=AND  UseBitMask=on  BitMask=bin2dec('0011111111111111')  BitMaskRealWorld=Stored Integer
  Bitwise Operator3 : simulink/Logic and Bit Operations/Bitwise Operator  logicop=NOT  UseBitMask=off  BitMask=bin2dec('0011111111111111')  BitMaskRealWorld=Stored Integer
  Bitwise Operator4 : simulink/Logic and Bit Operations/Bitwise Operator  logicop=OR  UseBitMask=off  NumInputPorts=2  BitMask=bin2dec('0011111111111111')  BitMaskRealWorld=Stored Integer
  Constant : Constant  Value=0.5
  Constant1 : Constant  Value=848
  Constant4 : Constant  Value=848
  Constant5 : Constant  Value=0.5
  Constant6 : Constant  OutDataTypeStr=uint16
  Data Type Conversion{,1..4} (5 alike) : DataTypeConversion  OutDataTypeStr=uint16
  Divide : Product  Inputs=*/
  Multiply : Product
  Shift Arithmetic1 : ArithShift  BitShiftNumber=2  BitShiftDirection=Left
  ACCToqReqValPV : Outport
  ToqReqVal : Outport  Port=2
  wires:
  Constant5/1 -> Divide/2
  Add/1 -> Divide/1
  Constant4/1 -> Add/2
  Data Type Conversion1/1 -> Add1/1
  Constant6/1 -> Add2/2
  Data Type Conversion/1 -> Multiply/2, Shift Arithmetic1/1
  Bitwise Operator2/1 -> Data Type Conversion1/1
  Bitwise Operator3/1 -> Add2/1
  Divide/1 -> Data Type Conversion/1
  Bitwise Operator4/1 -> Bitwise Operator2/1
  Bitwise Operator1/1 -> Data Type Conversion2/1
  Data Type Conversion2/1 -> Bitwise Operator3/1
  Shift Arithmetic1/1 -> Bitwise Operator4/1
  ACCToqReqVal/1 -> Add/1
  Add1/1 -> Bitwise Operator1/1
  ACCAlvRC/1 -> Data Type Conversion4/1
  Add2/1 -> ACCToqReqValPV/1
  ACCToqReqSts/1 -> Data Type Conversion3/1
  Data Type Conversion3/1 -> Bitwise Operator4/2
  Data Type Conversion4/1 -> Add1/2
  Constant/1 -> Multiply/1
  Multiply/1 -> Add3/1
  Constant1/1 -> Add3/2
  Add3/1 -> ToqReqVal/1

== system Intergration/TX/RADAR_HSC2_FrP00_0x242/Subsystem ==
  ACCAccReqVal : Inport
  ACCSysAlvRlngCtr : Inport  Port=2
  Add : Sum
  Add1 : Sum
  Add2 : Sum  Inputs=+-
  Bitwise Operator : simulink/Logic and Bit Operations/Bitwise Operator  logicop=AND  UseBitMask=on  BitMask=bin2dec('11111111')  BitMaskRealWorld=Stored Integer
  Bitwise Operator1 : simulink/Logic and Bit Operations/Bitwise Operator  logicop=AND  UseBitMask=on  BitMask=bin2dec('00000111')  BitMaskRealWorld=Stored Integer
  Bitwise Operator2 : simulink/Logic and Bit Operations/Bitwise Operator  logicop=AND  UseBitMask=on  BitMask=bin2dec('01111000')  BitMaskRealWorld=Stored Integer
  Constant : Constant  Value=0.005
  Constant1 : Constant  Value=7.22
  Constant2 : Constant  Value=7.22
  Constant3 : Constant  Value=0.005
  Data Type Conversion : DataTypeConversion  OutDataTypeStr=uint16
  Data Type Conversion1 : DataTypeConversion  OutDataTypeStr=uint16
  Data Type Conversion2 : DataTypeConversion  OutDataTypeStr=uint8
  Data Type Conversion3 : DataTypeConversion  OutDataTypeStr=uint8
  Data Type Conversion4 : DataTypeConversion  OutDataTypeStr=uint8
  Divide : Product  Inputs=*/
  Multiply : Product
  Shift Arithmetic1 : ArithShift  BitShiftNumber=8  BitShiftDirection=Right
  Shift Arithmetic2 : ArithShift  BitShiftNumber=3  BitShiftDirection=Left
  x242_byte0 : Outport
  x242_byte1 : Outport  Port=2
  AccReqVal : Outport  Port=3
  wires:
  ACCAccReqVal/1 -> Add/1
  Data Type Conversion/1 -> Multiply/1, Bitwise Operator/1
  Divide/1 -> Data Type Conversion1/1, Data Type Conversion/1
  Bitwise Operator/1 -> Data Type Conversion4/1
  Constant2/1 -> Add/2
  Add/1 -> Divide/1
  Constant3/1 -> Divide/2
  Data Type Conversion2/1 -> Shift Arithmetic2/1
  Bitwise Operator2/1 -> Add1/1
  Bitwise Operator1/1 -> Add1/2
  Add1/1 -> x242_byte0/1
  Shift Arithmetic2/1 -> Bitwise Operator2/1
  ACCSysAlvRlngCtr/1 -> Data Type Conversion2/1
  Data Type Conversion1/1 -> Shift Arithmetic1/1
  Shift Arithmetic1/1 -> Data Type Conversion3/1
  Constant/1 -> Multiply/2
  Multiply/1 -> Add2/1
  Constant1/1 -> Add2/2
  Add2/1 -> AccReqVal/1
  Data Type Conversion3/1 -> Bitwise Operator1/1
  Data Type Conversion4/1 -> x242_byte1/1

== system Intergration/TX/RADAR_HSC2_FrP00_0x242/Subsystem1 ==
  ACCAccReqSts : Inport
  ACCGoReq : Inport  Port=2
  Add : Sum
  Bitwise Operator : simulink/Logic and Bit Operations/Bitwise Operator  logicop=AND  UseBitMask=on  BitMask=bin2dec('01000000')  BitMaskRealWorld=Stored Integer
  Bitwise Operator1 : simulink/Logic and Bit Operations/Bitwise Operator  logicop=AND  UseBitMask=on  BitMask=bin2dec('00110000')  BitMaskRealWorld=Stored Integer
  Data Type Conversion1 : DataTypeConversion  OutDataTypeStr=uint8
  Data Type Conversion2 : DataTypeConversion  OutDataTypeStr=uint8
  Shift Arithmetic1 : ArithShift  BitShiftNumber=6  BitShiftDirection=Left
  Shift Arithmetic2 : ArithShift  BitShiftNumber=4  BitShiftDirection=Left
  x242_byte3 : Outport
  wires:
  Add/1 -> x242_byte3/1
  Bitwise Operator1/1 -> Add/2
  Bitwise Operator/1 -> Add/1
  Data Type Conversion1/1 -> Shift Arithmetic1/1
  Shift Arithmetic1/1 -> Bitwise Operator/1
  ACCGoReq/1 -> Data Type Conversion1/1
  Data Type Conversion2/1 -> Shift Arithmetic2/1
  Shift Arithmetic2/1 -> Bitwise Operator1/1
  ACCAccReqSts/1 -> Data Type Conversion2/1

== system Intergration/TX/RADAR_HSC2_FrP00_0x242/Subsystem2 ==
  ACCSysFltSts : Inport
  ACCSysSts_Radar : Inport  Port=2
  Add : Sum
  Bitwise Operator : simulink/Logic and Bit Operations/Bitwise Operator  logicop=AND  UseBitMask=on  BitMask=bin2dec('00111000')  BitMaskRealWorld=Stored Integer
  Bitwise Operator1 : simulink/Logic and Bit Operations/Bitwise Operator  logicop=AND  UseBitMask=on  BitMask=bin2dec('00000111')  BitMaskRealWorld=Stored Integer
  Data Type Conversion1 : DataTypeConversion  OutDataTypeStr=uint8
  Data Type Conversion2 : DataTypeConversion  OutDataTypeStr=uint8
  Shift Arithmetic1 : ArithShift  BitShiftNumber=3  BitShiftDirection=Left
  x242_byte5 : Outport
  wires:
  ACCSysFltSts/1 -> Data Type Conversion2/1
  Data Type Conversion2/1 -> Bitwise Operator1/1
  Bitwise Operator/1 -> Add/1
  Add/1 -> x242_byte5/1
  Bitwise Operator1/1 -> Add/2
  Data Type Conversion1/1 -> Shift Arithmetic1/1
  Shift Arithmetic1/1 -> Bitwise Operator/1
  ACCSysSts_Radar/1 -> Data Type Conversion1/1

== system Intergration/TX/RADAR_HSC2_FrP00_0x242/Subsystem3 ==
  ACCSdslReq_Radar : Inport
  Bitwise Operator2 : simulink/Logic and Bit Operations/Bitwise Operator  logicop=AND  UseBitMask=on  BitMask=bin2dec('10000000')  BitMaskRealWorld=Stored Integer
  Data Type Conversion2 : DataTypeConversion  OutDataTypeStr=uint8
  Shift Arithmetic1 : ArithShift  BitShiftNumber=7  BitShiftDirection=Left
  x242_byte6 : Outport
  wires:
  Bitwise Operator2/1 -> x242_byte6/1
  Shift Arithmetic1/1 -> Bitwise Operator2/1
  Data Type Conversion2/1 -> Shift Arithmetic1/1
  ACCSdslReq_Radar/1 -> Data Type Conversion2/1

== system Intergration/TX/RADAR_HSC2_FrP01_0x244/Subsystem10 ==
  AEBSysFltSts : Inport
  Bitwise Operator3 : simulink/Logic and Bit Operations/Bitwise Operator  logicop=AND  UseBitMask=on  BitMask=bin2dec('11100000')  BitMaskRealWorld=Stored Integer
  Data Type Conversion3 : DataTypeConversion  OutDataTypeStr=uint8
  Shift Arithmetic2 : ArithShift  BitShiftNumber=5  BitShiftDirection=Left
  x244_byte5 : Outport
  wires:
  AEBSysFltSts/1 -> Data Type Conversion3/1
  Shift Arithmetic2/1 -> Bitwise Operator3/1
  Data Type Conversion3/1 -> Shift Arithmetic2/1
  Bitwise Operator3/1 -> x244_byte5/1

== system Intergration/TX/RADAR_HSC2_FrP01_0x244/Subsystem5 ==
  AEBDclReqVal0 : Inport
  Add : Sum
  Add1 : Sum  Inputs=+-
  Bitwise Operator : simulink/Logic and Bit Operations/Bitwise Operator  logicop=AND  UseBitMask=on  BitMask=bin2dec('11111111')  BitMaskRealWorld=Stored Integer
  Constant : Constant  Value=12.7
  Constant1 : Constant  Value=0.1
  Constant4 : Constant  Value=0.1
  Constant5 : Constant  Value=12.7
  Data Type Conversion2 : DataTypeConversion  OutDataTypeStr=uint8
  Divide : Product  Inputs=*/  OutDataTypeStr=single
  Multiply : Product
  AEBDclReqVal : Outport
  x244_byte0 : Outport  Port=2
  wires:
  Data Type Conversion2/1 -> Bitwise Operator/1, Multiply/1
  Add/1 -> Divide/1
  Constant/1 -> Add/2
  Constant4/1 -> Multiply/2
  Divide/1 -> Data Type Conversion2/1
  Add1/1 -> AEBDclReqVal/1
  Multiply/1 -> Add1/1
  Constant5/1 -> Add1/2
  Constant1/1 -> Divide/2
  AEBDclReqVal0/1 -> Add/1
  Bitwise Operator/1 -> x244_byte0/1

== system Intergration/TX/RADAR_HSC2_FrP01_0x244/Subsystem6 ==
  AEBPrflReq : Inport
  Add : Sum
  Bitwise Operator1 : simulink/Logic and Bit Operations/Bitwise Operator  logicop=AND  UseBitMask=on  BitMask=bin2dec('01111111')  BitMaskRealWorld=Stored Integer
  Bitwise Operator2 : simulink/Logic and Bit Operations/Bitwise Operator  logicop=AND  UseBitMask=on  BitMask=bin2dec('10000000')  BitMaskRealWorld=Stored Integer
  Constant : Constant  Value=0  OutDataTypeStr=uint8
  Data Type Conversion2 : DataTypeConversion  OutDataTypeStr=uint8
  Shift Arithmetic1 : ArithShift  BitShiftNumber=7  BitShiftDirection=Left
  x244_byte1 : Outport
  wires:
  Data Type Conversion2/1 -> Shift Arithmetic1/1
  Shift Arithmetic1/1 -> Bitwise Operator2/1
  AEBPrflReq/1 -> Data Type Conversion2/1
  Bitwise Operator2/1 -> Add/2
  Constant/1 -> Bitwise Operator1/1
  Add/1 -> x244_byte1/1
  Bitwise Operator1/1 -> Add/1

== system Intergration/TX/RADAR_HSC2_FrP01_0x244/Subsystem7 ==
  ACCAEBBrkJerkLvlReq : Inport
  AEBSysSts : Inport  Port=2
  Add : Sum
  Bitwise Operator1 : simulink/Logic and Bit Operations/Bitwise Operator  logicop=AND  UseBitMask=on  BitMask=bin2dec('11100000')  BitMaskRealWorld=Stored Integer
  Bitwise Operator2 : simulink/Logic and Bit Operations/Bitwise Operator  logicop=AND  UseBitMask=on  BitMask=bin2dec('00011100')  BitMaskRealWorld=Stored Integer
  Data Type Conversion1 : DataTypeConversion  OutDataTypeStr=uint8
  Data Type Conversion2 : DataTypeConversion  OutDataTypeStr=uint8
  Shift Arithmetic1 : ArithShift  BitShiftNumber=2  BitShiftDirection=Left
  Shift Arithmetic2 : ArithShift  BitShiftNumber=5  BitShiftDirection=Left
  x244_byte2 : Outport
  wires:
  Shift Arithmetic1/1 -> Bitwise Operator2/1
  Shift Arithmetic2/1 -> Bitwise Operator1/1
  Add/1 -> x244_byte2/1
  AEBSysSts/1 -> Data Type Conversion1/1
  ACCAEBBrkJerkLvlReq/1 -> Data Type Conversion2/1
  Data Type Conversion2/1 -> Shift Arithmetic1/1
  Data Type Conversion1/1 -> Shift Arithmetic2/1
  Bitwise Operator2/1 -> Add/1
  Bitwise Operator1/1 -> Add/2

== system Intergration/TX/RADAR_HSC2_FrP01_0x244/Subsystem8 ==
  AEBDclReqSts : Inport
  AEBPedtrnSysSts : Inport  Port=2
  AEBHydBrkAstLvlReq : Inport  Port=3
  Add : Sum  Inputs=+++
  Bitwise Operator1 : simulink/Logic and Bit Operations/Bitwise Operator  logicop=AND  UseBitMask=on  BitMask=bin2dec('00011100')  BitMaskRealWorld=Stored Integer
  Bitwise Operator2 : simulink/Logic and Bit Operations/Bitwise Operator  logicop=AND  UseBitMask=on  BitMask=bin2dec('00000011')  BitMaskRealWorld=Stored Integer
  Bitwise Operator3 : simulink/Logic and Bit Operations/Bitwise Operator  logicop=AND  UseBitMask=on  BitMask=bin2dec('11100000')  BitMaskRealWorld=Stored Integer
  Data Type Conversion1 : DataTypeConversion  OutDataTypeStr=uint8
  Data Type Conversion2 : DataTypeConversion  OutDataTypeStr=uint8
  Data Type Conversion3 : DataTypeConversion  OutDataTypeStr=uint8
  Shift Arithmetic1 : ArithShift  BitShiftNumber=2  BitShiftDirection=Left
  Shift Arithmetic2 : ArithShift  BitShiftNumber=5  BitShiftDirection=Left
  x244_byte3 : Outport
  wires:
  Bitwise Operator3/1 -> Add/1
  Shift Arithmetic1/1 -> Bitwise Operator1/1
  Bitwise Operator1/1 -> Add/3
  Data Type Conversion2/1 -> Bitwise Operator2/1
  Data Type Conversion3/1 -> Shift Arithmetic2/1
  Add/1 -> x244_byte3/1
  Shift Arithmetic2/1 -> Bitwise Operator3/1
  Bitwise Operator2/1 -> Add/2
  Data Type Conversion1/1 -> Shift Arithmetic1/1
  AEBDclReqSts/1 -> Data Type Conversion2/1
  AEBHydBrkAstLvlReq/1 -> Data Type Conversion3/1
  AEBPedtrnSysSts/1 -> Data Type Conversion1/1
